simulink model "Q3"  (R2020b)
settings: Solver=VariableStepAuto  StartTime=0.0  StopTime=10.0  RelTol=1e-3
model workspace (MAT data in the model file):
  Ki = Simulink.Parameter
  Ki.Value = 40
  Ki.DataType = 'auto'
  Ki.Dimensions = [1 1]
  Kp = Simulink.Parameter
  Kp.Value = 5000
  Kp.DataType = 'auto'
  Kp.Dimensions = [1 1]
  b = Simulink.Parameter
  b.Value = 50
  b.DataType = 'auto'
  b.Dimensions = [1 1]
  m = Simulink.Parameter
  m.Value = 1000
  m.DataType = 'auto'
  m.Dimensions = [1 1]
  u = Simulink.Parameter
  u.Value = 500
  u.DataType = 'auto'
  u.Dimensions = [1 1]
values from neighbouring files (symbols this model uses):
  b = 50.0    [datadic2.sldd]
  Ki = 40.0    [datadic2.sldd]
  Kp = 5000.0    [datadic2.sldd]
  m = 1000.0    [datadic2.sldd]
settings Model: Creator=DELL  LastModifiedBy=DELL

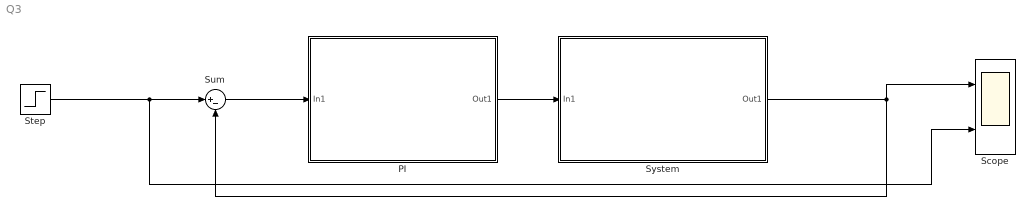
== system Q3 ==
  PI : Subsystem
  Scope : Scope  NumInputPorts=2
  Step : Step  After=u  SampleTime=0
  Sum : Sum  Inputs=|+-
  System : Subsystem
  wires:
  System/1(Out1) -> Sum/2, Scope/1
  PI/1(Out1) -> System/1(In1)
  Sum/1 -> PI/1(In1)
  Step/1 -> Scope/2, Sum/1

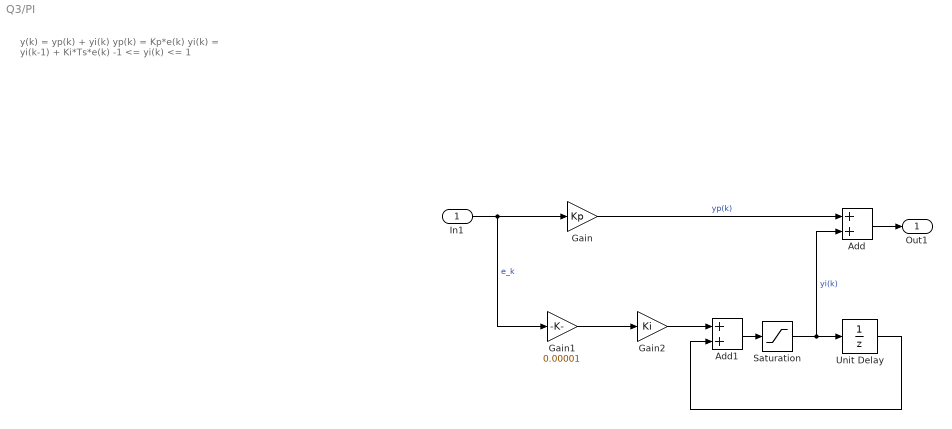
== system Q3/PI ==
  note: y(k) = yp(k) + yi(k)
      | yp(k) = Kp*e(k)
      | yi(k) = yi(k-1) + Ki*Ts*e(k)
      | -1 <= yi(k) <= 1
  In1 : Inport
  Add : Sum
  Add1 : Sum
  Gain : Gain  Gain=Kp
  Gain1 : Gain  Gain=0.00001
  Gain2 : Gain  Gain=Ki
  Saturation : Saturate  UpperLimit=1  LowerLimit=-1
  Unit Delay : UnitDelay  SampleTime=-1  HasFrameUpgradeWarning=on
  Out1 : Outport
  wires:
  Add/1 -> Out1/1
  Gain/1 -> Add/1  "yp(k)"
  Saturation/1 -> Add/2, Unit Delay/1  "yi(k)"
  Add1/1 -> Saturation/1
  Gain2/1 -> Add1/1
  In1/1 -> Gain1/1, Gain/1  "e_k"
  Gain1/1 -> Gain2/1
  Unit Delay/1 -> Add1/2

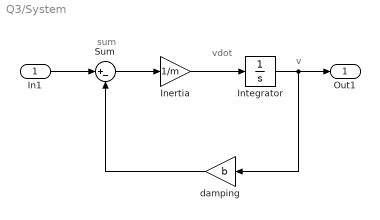
== system Q3/System ==
  note: vdot
  note: sum
  note: v
  In1 : Inport
  Inertia : Gain  Gain=1/m
  Integrator : Integrator
  Sum : Sum  Inputs=|+-
  damping : Gain  Gain=b
  Out1 : Outport
  wires:
  In1/1 -> Sum/1
  Sum/1 -> Inertia/1
  Inertia/1 -> Integrator/1
  damping/1 -> Sum/2
  Integrator/1 -> Out1/1, damping/1
